simulink model "WithLoad_Simple"  (R2017b)
settings: Solver=ode3  StartTime=0.0  StopTime=10  FixedStep=0.005  RelTol=1e-3  EnableMultiTasking=on
libraries: mblibv1 x61
(part 3 of 3)

== matlab function WithLoad_Simple/Target_Momentum ==
  data: mt input; It input; Px output; rx input; ry input; vx input; vy input; wz input; Py output; L output
function [Px,Py,L] = Target_Momentum(mt,It,rx,ry,vx,vy,wz)
%#eml

Px = mt*vx;
Py = mt*vy;
L  = It*wz + mt*(rx*vy - ry*vx);
end

== matlab function WithLoad_Simple/SpaceRobotic_Blue_Dynamics/Force ==
  data: counter input; F output; omega input; It input
function F = Force(counter,omega,It)
%#eml

F = [0;0;0;0;0;0];   
if( counter ==10)
    F = [0;0;omega*It/0.005;0;0;0]; 
else 
    F = [0;0;0;0;0;0]; 
end
end
